simulink model "Active_Suspension_Control_NC"  (R2012b)
settings: Solver=ode45  StartTime=0.0  StopTime=18  RelTol=1e-3
values from neighbouring files (symbols this model uses):
  Ad = [0.978483123139 0 0 -1.68493497681 0 0 0 0.897751924192 0 0 -7.27611115986 0 ... (36 elements, 6x6)]    [Active_Suspension_Control_Model.mat]
  Bdu = [-0.00672402401896 0.0114116156036 -0.0288308554725 -0.526542180252 0.812065977663 -1.91495958182 -0.00672402401896 0.0114116156036 0.0288308554725 -0.526542180252 0.812065977663 1.91495958182 ... (24 elements, 6x4)]    [Active_Suspension_Control_Model.mat]
  Bdw = [-0.00537921921517 0.00912929248288 -0.023064684378 -0.421233744202 0.649652782131 -1.53196766546 -0.00537921921517 0.00912929248288 0.023064684378 -0.421233744202 0.649652782131 1.53196766546 ... (48 elements, 6x8)]    [Active_Suspension_Control_Model.mat]
  Cd = [-71.5883668904 0 0 0 -404.102013423 0 0 0 -659.758389262 -4.26666666667 0 0 ... (18 elements, 3x6)]    [Active_Suspension_Control_Model.mat]
  Dd = [-22.3713646532 45.1006711409 -128.859060403 -22.3713646532 45.1006711409 128.859060403 -22.3713646532 -45.1006711409 -128.859060403 -22.3713646532 -45.1006711409 128.859060403 ... (36 elements, 3x12)]    [Active_Suspension_Control_Model.mat]
settings Model: Creator=koenigg  LastModifiedBy=juanj
settings DataIOCC: MaxDataPoints=10000  SignalLoggingSaveFormat=ModelDataLogs  OutputOption=SpecifiedOutputTimes  OutputTimes=[0:.005:3600*.005-.01]'
settings OptimizationCC: ExpressionDepthLimit=128
settings DebuggingCC: MultiTaskDSMMsg=warning  MultiTaskCondExecSysMsg=none
settings RTWCC: IncludeERTFirstTime=on
settings CodeAppCC: CustomSymbolStrType=$N$R$M_T  InternalIdentifier=Shortened

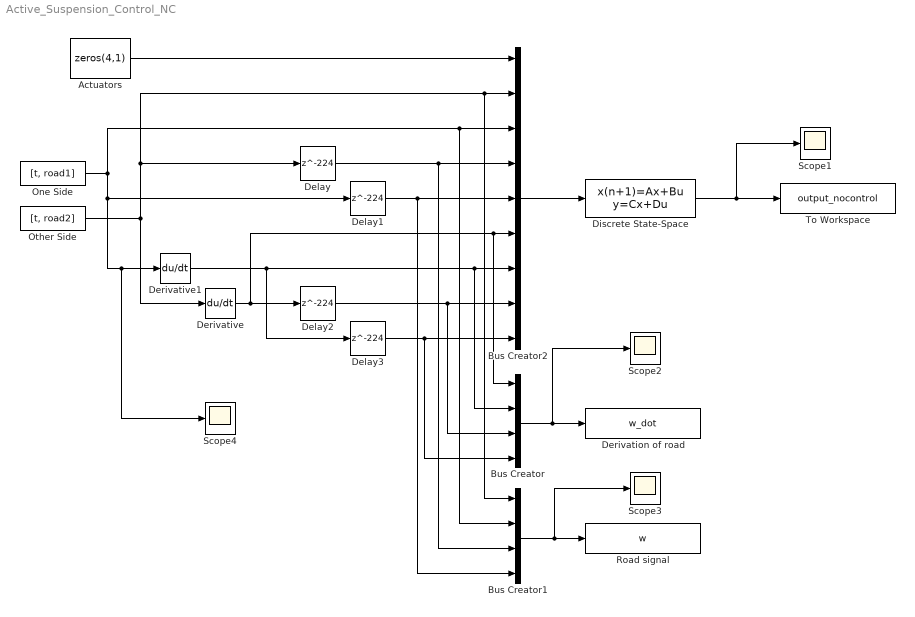
== system Active_Suspension_Control_NC ==
  Actuators : Constant  Value=zeros(4,1)
  Bus Creator : BusCreator
  Bus Creator1 : BusCreator
  Bus Creator2 : BusCreator  Inputs=9
  Delay{,1..3} (4 alike) : Delay  DelayLength=224  SampleTime=.005
  Derivation of road : ToWorkspace  VariableName=w_dot  SampleTime=-1  SaveFormat=Timeseries
  Derivative : Derivative
  Derivative1 : Derivative
  Discrete State-Space : DiscreteStateSpace  A=Ad  B=[Bdu Bdw]  C=Cd  D=Dd  SampleTime=.005
  One Side : FromWorkspace  VariableName=[t, road1]  SampleTime=0
  Other Side : FromWorkspace  VariableName=[t, road2]  SampleTime=0
  Road signal : ToWorkspace  VariableName=w  SampleTime=-1  SaveFormat=Timeseries
  Scope{1..4} (4 alike) : Scope
      Scope1 settings: TickLabels=on  ShowLegends=on  TimeRange=20
      Scope2 settings: TickLabels=on  ShowLegends=on  TimeRange=15
      Scope3 settings: TickLabels=on  ShowLegends=on  TimeRange=20  SaveName=ScopeData2
      Scope4 settings: TickLabels=on  ShowLegends=on  TimeRange=15  SaveName=ScopeData3
  To Workspace : ToWorkspace  VariableName=output_nocontrol  SampleTime=-1  SaveFormat=Timeseries
  wires:
  Bus Creator2/1 -> Discrete State-Space/1
  Actuators/1 -> Bus Creator2/1
  Other Side/1 -> Derivative/1, Delay/1, Bus Creator1/1, Bus Creator2/2
  Delay1/1 -> Bus Creator1/4, Bus Creator2/5
  Delay/1 -> Bus Creator1/3, Bus Creator2/4
  Derivative/1 -> Delay2/1, Bus Creator/1, Bus Creator2/6
  Delay3/1 -> Bus Creator/4, Bus Creator2/9
  Delay2/1 -> Bus Creator/3, Bus Creator2/8
  One Side/1 -> Delay1/1, Scope4/1, Derivative1/1, Bus Creator1/2, Bus Creator2/3
  Derivative1/1 -> Delay3/1, Bus Creator/2, Bus Creator2/7
  Bus Creator/1 -> Scope2/1, Derivation of road/1
  Bus Creator1/1 -> Scope3/1, Road signal/1
  Discrete State-Space/1 -> Scope1/1, To Workspace/1
